simulink library "NFSModelsLibrary"  (R2020a)
settings: Solver=VariableStepAuto  StartTime=0.0  StopTime=10.0  RelTol=1e-3
undefined symbols (not defined in the file or in its folder): Earth, F, Light, MIL, Newton, nfs, Raphson, sigbuilder_block, WGS84
libraries: sharedutil x3, simulink x2, ModelsLibrary x2, $bdroot x2, aerolibwind2 x2, aerolibtransform2 x1
(part 1 of 3)
settings Model: Creator=AHKh  LastModifiedBy=AHKh
settings DataIOCC: ReturnWorkspaceOutputs=off
settings DebuggingCC: ArithmeticOperatorsInVariantConditions=warning
settings SFSimCC: SimUseLocalCustomCode=off  CustomCodeUndefinedFunction=UseInterfaceOnly
settings RTWCC: RTWUseLocalCustomCode=off
settings CodeAppCC: StateflowObjectComments=on

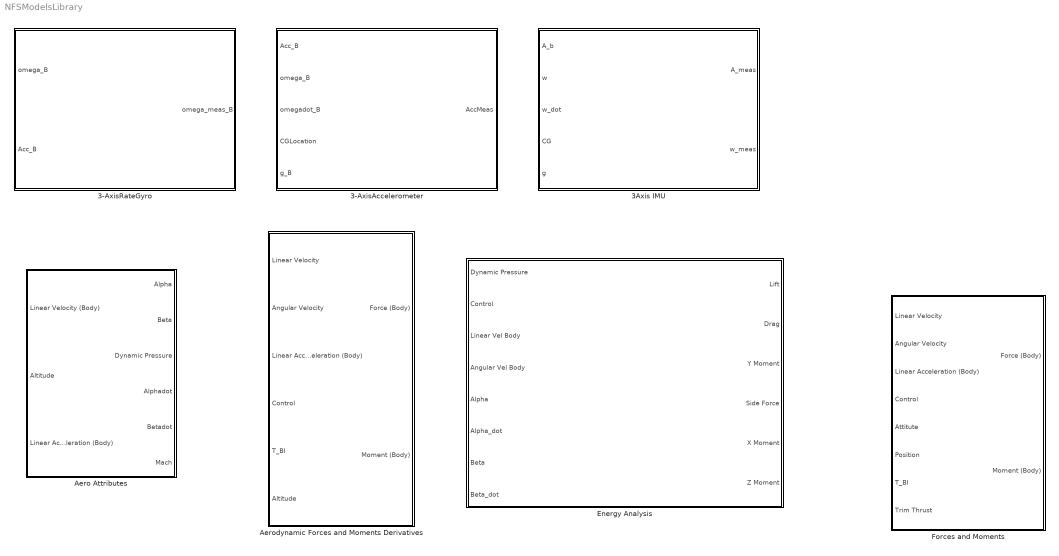
== system NFSModelsLibrary ==
  3-AxisAccelerometer : Subsystem  mask{units=Metric (MKS), SensorLoc=[0; 0; 0], gtype=off, dtype_a=on, w_a=190, z_a=0.707, SFCC=eye(3), SensorBias=[0; 0; 0], Ts=0.001, AccNoiseCheck=on, NoiseSeeds=[23093; 23094; 23095], NoisePower=[0.001; 0.001; 0.001], satUpper=[inf; inf; inf], satLower=[-inf; -inf; -inf]}
      mask prompts: units "Unit"; SensorLoc "Accelerometer Location"; gtype "Subtracting Gravity"; dtype_a "Considering 2nd-Order Dynamics"; w_a "Natural Frequency (rad/s)"; z_a "Damping Ratio"; SFCC "Scale Factor and Cross-Coupling"; SensorBias "Measurment Bias"; Ts "Update Rate (sec)"; AccNoiseCheck "Considering Noise"; NoiseSeeds "Noise Seeds"; NoisePower "Noise Power"; satUpper "Output Upper Limits"; satLower "Output Lower Limits"
      mask TypeOptions units: Metric (MKS)
      mask DialogControl DescGroupVar Prompt: Three-Axis Accelerometer
      mask DialogControl DescTextVar Prompt: Implements a three-axis accelerometer
      mask DialogControl Container4 Prompt: Main
      mask DialogControl units Tooltip: Metric System of Units
      mask DialogControl Container5 Prompt: Noise Characteristics
      mask Display:
      | port_label('input',1,'[Acc]^{B}_B (m/s^2)','texmode','on');
      | port_label('input',2,'[\omega]^B_B (rad/s)','texmode','on');
      | port_label('input',3,'[d\omega/dt]^B_B (rad/s^2)','texmode','on');
      | port_label('input',4,'[CG]^B_B (m)','texmode','on');
      | port_label('input',5,'[g]^B_B (m/s^2)','texmode','on');
      | port_label('output',1,'[Acc_{meas}]^{B}_B (m/s^2)','texmode','on');
  3-AxisRateGyro : Subsystem  mask(Three-Axis Rate Gyroscope){dtype_g=on, w_g=190, z_g=0.707, SFCC=eye(3), SensorBias=[0; 0; 0], gSensitivity=[0; 0; 0], Ts=0.001, GyroNoiseCheck=on, NoiseSeeds=[23093; 23094; 23095], NoisePower=[0.0001; 0.0001; 0.0001], satUpper=[inf; inf; inf], satLower=[-inf; -inf; -inf]}
      mask prompts: dtype_g "Considering 2nd-Order Dynamics"; w_g "Natural Frequency (rad/s)"; z_g "Damping Ratio"; SFCC "Scale Factors and Cross-Coupling"; SensorBias "Measurment Bias"; gSensitivity "G-Sensitive Bias"; Ts "Update Rate (sec)"; GyroNoiseCheck "Considering Noise"; NoiseSeeds "Noise Seeds"; NoisePower "Noise Power"; satUpper "Output Upper Bound"; satLower "Output Lower Bound"
      mask DialogControl DescGroupVar Prompt: Three-Axis Gyroscope
      mask DialogControl DescTextVar Prompt: Implements a three-axis gyroscope.
      mask DialogControl Container4 Prompt: Main
      mask DialogControl Container5 Prompt: Noise Characteristics
      mask Display:
      | port_label('input',1,'[\omega]^B_B (rad/s)','texmode','on');
      | port_label('input',2,'[Acc]^{B}_B (m/s^2)','texmode','on');
      | port_label('output',1,'[\omega_{meas}]^{B}_B (rad/s)','texmode','on');
  3Axis IMU : Subsystem  mask{units=Metric (MKS), IMULocation=[0; 0; 0], Ts=0.001, AccSubtractGravity=off, dtype_a=on, AccNaturalFrequency=190, AccDampingRatio=0.707, AccSFCC=eye(3), AccMeasurmentBias=[0; 0; 0], AccMeasUpperLimit=[inf; inf; inf], AccMeasLowerLimit=[-inf; -inf; -inf], AccNoiseCheck=on, AccNoiseSeeds=[23093; 23094; 23095], AccNoisePower=[0.0001; 0.0001; 0.0001], dtype_g=on, GyroNaturalFrequency=190, GyroDampingRatio=0.707, GyroSFCC=eye(3), GyroMeasurmentBias=[0; 0; 0], GyroGSensitiveBias=[0; 0; 0], GyroMeasUpperLimit=[inf; inf; inf], GyroMeasLowerLimit=[-inf; -inf; -inf], GyroNoiseCheck=on, GyroNoiseSeeds=[23093; 23094; 23095], GyroNoisePower=[0.0001; 0.0001; 0.0001]}
      mask prompts: IMULocation "IMU Location (m)"; Ts "Update Rate (sec)"; AccSubtractGravity "Subtracting Gravity"; dtype_a "Considering 2nd-Order Dynamics"; AccNaturalFrequency "Natural Frequency (rad/s)"; AccDampingRatio "Damping Ratio"; AccSFCC "Scale Factor and Cross Coupling"; AccMeasurmentBias "Measurment Bias"; AccMeasUpperLimit "Measurment Upper Limit"; AccMeasLowerLimit "Measurment Lower Limit"; AccNoiseCheck "Considering Noise"; AccNoiseSeeds "Noise Seeds"; AccNoisePower "Noise Power"; dtype_g "Considering 2nd-Order Dynamics"; GyroNaturalFrequency "Natural Frequency (rad/s)"; GyroDampingRatio "Damping Ratio"; GyroSFCC "Scale Factor and Cross Coupling"; GyroMeasurmentBias "Measurment Bias"; GyroGSensitiveBias "G-Sensitive Bias"; GyroMeasUpperLimit "Measurment Upper Limit"; GyroMeasLowerLimit "Measurment Lower Limit"; GyroNoiseCheck "Considering Noise"; GyroNoiseSeeds "Noise Seeds"; GyroNoisePower "Noise Power"
      mask init:
      | a1 = get(gcbh,'AccSubtractGravity');
      | a2 = get(gcbh,'dtype_a');
      | a3 = get(gcbh,'AccNoiseCheck');
      | a4 = get(gcbh,'dtype_g');
      | a5 = get(gcbh,'GyroNoiseCheck');
      | Acc = getSimulinkBlockHandle([gcb '/3-AxisAccelerometer']);
      | Gyro = getSimulinkBlockHandle([gcb '/3-AxisRateGyro']);
      | set(Acc,'gtype',a1);
      | set(Acc,'dtype_a',a2);
      | set(Acc,'AccNoiseCheck',a3);
      | set(Gyro,'dtype_g',a4);
      | set(Gyro,'GyroNoiseCheck',a5);
      mask TypeOptions units: Metric (MKS)
      mask DialogControl DescGroupVar Prompt: 3-Axis IMU
      mask DialogControl DescTextVar Prompt: Implements 3-axis Inertial Measurment Unit (IMU)
      mask DialogControl Container4 Prompt: Main
      mask DialogControl Container9 Prompt: Accelerometer
      mask DialogControl Container11 Prompt: Accelerometer General
      mask DialogControl Container14 Prompt: Accelerometer Noise
      mask DialogControl Container5 Prompt: Gyroscope
      mask DialogControl Container7 Prompt: Gyroscope General
      mask DialogControl Container8 Prompt: Gyroscope Noise
      mask Display:
      | port_label('input',1,'[Acc]^{B}_B (m/s^2)','texmode','on');
      | port_label('input',2,'[\omega]^B_B (rad/s)','texmode','on');
      | port_label('input',3,'[d\omega/dt]^B_B (rad/s^2)','texmode','on');
      | port_label('input',4,'[CG]^B_B (m)','texmode','on');
      | port_label('input',5,'[g]^B_B (m/s^2)','texmode','on');
      | port_label('output',1,'[Acc_{meas}]^{B}_B (m/s^2)','texmode','on');
      | port_label('output',2,'[\omega_{meas}]^{B}_B (rad/s)','texmode','on');
  Aero Attributes : Subsystem
  Aerodynamic Forces and Moments Derivatives : Subsystem
  Energy Analysis : Subsystem  mask{ae=nfs}
      mask prompts: ae "Aero Coefficients"
  Forces and Moments : Subsystem

== system NFSModelsLibrary/3-AxisAccelerometer ==
  Acc_B : Inport  Unit=m/s^2  PortDimensions=[3,1]
  omega_B : Inport  Port=2  Unit=rad/s  PortDimensions=[3,1]
  omegadot_B : Inport  Port=3  Unit=rad/s^2  PortDimensions=[3,1]
  CGLocation : Inport  Port=4  Unit=m  PortDimensions=[3,1]
  g_B : Inport  Port=5  Unit=m/s^2  PortDimensions=[3,1]
  Accelerometer Dynamic : Subsystem
  Gain : Gain  Gain=[1 -1 1]'  SaturateOnIntegerOverflow=on  OutDataTypeStr=Inherit: Same as input  ParamDataTypeStr=Inherit: Same as input
  Measurement bias : Constant  Value=SensorBias
  Noise Check : Subsystem
  Product : Product  Multiplication=Matrix(*)  SaturateOnIntegerOverflow=on  OutDataTypeStr=Inherit: Same as first input
  Random bias : simulink/Sources/Band-Limited White Noise  Cov=NoisePower  Ts=Ts  seed=NoiseSeeds
  Reshape : Reshape  OutputDimensionality=Column vector (2-D)
  Reshape1 : Reshape
  Saturation : Saturate  UpperLimit=satUpper  LowerLimit=satLower
  Scale factors & Cross-coupling errors : Constant  Value=SFCC
  Sum1 : Sum  Inputs=|++  SaturateOnIntegerOverflow=on
  Sum2 : Sum  Inputs=|+-
  Sum3 : Sum  Inputs=|++
  Sum4 : Sum  Inputs=++|  SaturateOnIntegerOverflow=on
  Sum5 : Sum  Inputs=|++
  Sum7 : Sum  Inputs=|+-  SaturateOnIntegerOverflow=on
  w x (w x d) : Subsystem
  wdot x d : sharedutil/3x3 Cross Product
      settings: SourceProductBaseCode=AE,PW,MT,VE,VP
  wl_ins : Constant  Value=SensorLoc
  AccMeas : Outport  Unit=m/s^2  PortDimensions=[3,1]  VectorParamsAs1DForOutWhenUnconnected=off
  wires:
  Gain/1 -> w x (w x d)/2(CGAccdistance), wdot x d/2
  Sum4/1 -> Accelerometer Dynamic/1(AccIn)
  omegadot_B/1 -> wdot x d/1
  omega_B/1 -> w x (w x d)/1(omega_B)
  Scale factors & Cross-coupling errors/1 -> Product/1
  Measurement bias/1 -> Sum4/2
  Sum7/1 -> Gain/1
  wdot x d/1 -> Sum5/2
  CGLocation/1 -> Sum7/1
  Accelerometer Dynamic/1("AccOut ") -> Sum1/1
  Saturation/1 -> AccMeas/1
  Product/1 -> Reshape1/1
  Sum1/1 -> Saturation/1
  Random bias/1 -> Noise Check/1(NoiseIn)
  Reshape1/1 -> Sum4/1
  Sum5/1 -> Product/2
  Acc_B/1 -> Sum2/1
  g_B/1 -> Sum2/2
  Sum2/1 -> Sum3/1
  w x (w x d)/1(w x ( w x d)) -> Sum3/2
  Sum3/1 -> Sum5/1
  wl_ins/1 -> Reshape/1
  Reshape/1 -> Sum7/2
  Noise Check/1("NoiseOut ") -> Sum1/2

== system NFSModelsLibrary/3-AxisRateGyro ==
  omega_B : Inport  Unit=rad/s  PortDimensions=3
  Acc_B : Inport  Port=2  Unit=m/s^2  PortDimensions=3
  Gravity : Constant  Value=9.806
  Gyroscope Dynamic : Subsystem
  Measurement bias : Constant  Value=SensorBias
  Noise Check : Subsystem
  Product : Product  Multiplication=Matrix(*)  SaturateOnIntegerOverflow=on  OutDataTypeStr=Inherit: Same as first input
  Product1 : Product  SaturateOnIntegerOverflow=on  OutDataTypeStr=Inherit: Same as first input
  Product2 : Product  Inputs=*/  SaturateOnIntegerOverflow=on  OutDataTypeStr=Inherit: Same as first input
  Random bias : simulink/Sources/Band-Limited White Noise  Cov=NoisePower  Ts=Ts  seed=NoiseSeeds
  Saturation : Saturate  UpperLimit=satUpper  LowerLimit=satLower
  "Scale factors & Cross-coupling errors " : Constant  Value=SFCC
  Sum1 : Sum  Inputs=|++  SaturateOnIntegerOverflow=on
  Sum4 : Sum  Inputs=+++  SaturateOnIntegerOverflow=on
  g-sensitive bias : Constant  Value=gSensitivity
  omega_meas_B : Outport  Unit=rad/s  VectorParamsAs1DForOutWhenUnconnected=off
  wires:
  Product/1 -> Sum4/1
  Gyroscope Dynamic/1(pqr Out) -> Sum1/1
  Acc_B/1 -> Product2/1
  Product2/1 -> Product1/1
  Sum1/1 -> Saturation/1
  omega_B/1 -> Product/2
  Random bias/1 -> Noise Check/1(NoiseIn)
  Saturation/1 -> omega_meas_B/1
  Measurement bias/1 -> Sum4/2
  "Scale factors & Cross-coupling errors "/1 -> Product/1
  Sum4/1 -> Gyroscope Dynamic/1(pqr In)
  g-sensitive bias/1 -> Product1/2
  Product1/1 -> Sum4/3
  Gravity/1 -> Product2/2
  Noise Check/1("NoiseOut ") -> Sum1/2

== system NFSModelsLibrary/3Axis IMU ==
  A_b : Inport  Unit=m/s^2  PortDimensions=[3,1]
  w : Inport  Port=2  Unit=rad/s  PortDimensions=[3,1]
  w_dot : Inport  Port=3  Unit=rad/s^2  PortDimensions=[3,1]
  CG : Inport  Port=4  Unit=m  PortDimensions=[3,1]
  g : Inport  Port=5  Unit=m/s^2  PortDimensions=[3,1]
  3-AxisAccelerometer : ModelsLibrary/3-AxisAccelerometer  units=Metric (MKS)  SensorLoc=IMULocation  gtype=off  dtype_a=on  w_a=AccNaturalFrequency  z_a=AccDampingRatio  SFCC=AccSFCC  SensorBias=AccMeasurmentBias  Ts=Ts  AccNoiseCheck=on  NoiseSeeds=AccNoiseSeeds  NoisePower=AccNoisePower  satUpper=AccMeasUpperLimit  satLower=AccMeasLowerLimit
  3-AxisRateGyro : ModelsLibrary/3-AxisRateGyro  dtype_g=on  w_g=GyroNaturalFrequency  z_g=GyroDampingRatio  SFCC=GyroSFCC  SensorBias=GyroMeasurmentBias  gSensitivity=GyroGSensitiveBias  Ts=Ts  GyroNoiseCheck=on  NoiseSeeds=GyroNoiseSeeds  NoisePower=GyroNoisePower  satUpper=GyroMeasUpperLimit  satLower=GyroMeasLowerLimit
  A_meas : Outport  Unit=m/s^2  PortDimensions=[3,1]  VectorParamsAs1DForOutWhenUnconnected=off
  w_meas : Outport  Port=2  Unit=rad/s  PortDimensions=[3,1]  VectorParamsAs1DForOutWhenUnconnected=off
  wires:
  3-AxisRateGyro/1 -> w_meas/1
  w/1 -> 3-AxisRateGyro/1, 3-AxisAccelerometer/2
  A_b/1 -> 3-AxisRateGyro/2, 3-AxisAccelerometer/1
  3-AxisAccelerometer/1 -> A_meas/1
  w_dot/1 -> 3-AxisAccelerometer/3
  CG/1 -> 3-AxisAccelerometer/4
  g/1 -> 3-AxisAccelerometer/5

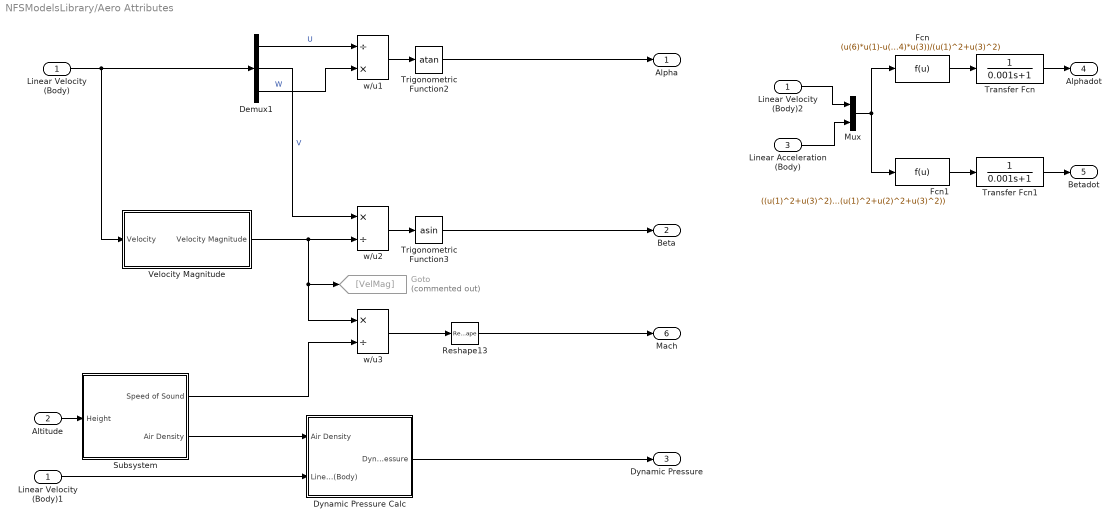
== system NFSModelsLibrary/Aero Attributes ==
  Linear Velocity (Body) : Inport  PortDimensions=[3,1]
  Altitude : Inport  Port=2
  Linear Acceleration (Body) : Inport  Port=3  PortDimensions=[3,1]
  Demux1 : Demux  Outputs=3
      settings: DisplayOption=none
  Dynamic Pressure Calc : Subsystem
  Fcn : Fcn  Expr=(u(6)*u(1)-u(4)*u(3))/(u(1)^2+u(3)^2)
  Fcn1 : Fcn  Expr=((u(1)^2+u(3)^2)*u(5)-u(2)*(u(1)*u(4)+u(3)*u(6)))/(sqrt(u(1)^2+u(3)^2)*(u(1)^2+u(2)^2+u(3)^2))
  Goto : Goto  Commented=on  GotoTag=VelMag
  Linear Velocity (Body)1 : InportShadow  PortDimensions=[3,1]
  Linear Velocity (Body)2 : InportShadow  PortDimensions=[3,1]
  Mux : Mux  Inputs=2
  Reshape13 : Reshape
  Subsystem : Subsystem
  Transfer Fcn : TransferFcn  Denominator=[0.001 1]
  Transfer Fcn1 : TransferFcn  Denominator=[0.001 1]
  Trigonometric Function2 : Trigonometry  Operator=atan
  Trigonometric Function3 : Trigonometry  Operator=asin
  Velocity Magnitude : Subsystem
  w/u1 : Product  Inputs=/*  InputSameDT=on  SaturateOnIntegerOverflow=on  OutDataTypeStr=Inherit: Same as first input
  w/u2 : Product  Inputs=*/  InputSameDT=on  SaturateOnIntegerOverflow=on  OutDataTypeStr=Inherit: Same as first input
  w/u3 : Product  Inputs=*/  InputSameDT=on  SaturateOnIntegerOverflow=on  OutDataTypeStr=Inherit: Same as first input
  Alpha : Outport  VectorParamsAs1DForOutWhenUnconnected=off
  Beta : Outport  Port=2  VectorParamsAs1DForOutWhenUnconnected=off
  Dynamic Pressure : Outport  Port=3  VectorParamsAs1DForOutWhenUnconnected=off
  Alphadot : Outport  Port=4  VectorParamsAs1DForOutWhenUnconnected=off
  Betadot : Outport  Port=5  VectorParamsAs1DForOutWhenUnconnected=off
  Mach : Outport  Port=6  VectorParamsAs1DForOutWhenUnconnected=off
  wires:
  Fcn1/1 -> Transfer Fcn1/1
  Fcn/1 -> Transfer Fcn/1
  Mux/1 -> Fcn/1, Fcn1/1
  Linear Acceleration (Body)/1 -> Mux/2
  Linear Velocity (Body)2/1 -> Mux/1
  Linear Velocity (Body)/1 -> Demux1/1, Velocity Magnitude/1(Velocity)
  Demux1/1 -> w/u1/1  "U"
  Demux1/2 -> w/u2/1  "V"
  Demux1/3 -> w/u1/2  "W"
  w/u1/1 -> Trigonometric Function2/1
  w/u2/1 -> Trigonometric Function3/1
  Trigonometric Function2/1 -> Alpha/1
  w/u3/1 -> Reshape13/1
  Altitude/1 -> Subsystem/1(Height)
  Linear Velocity (Body)1/1 -> Dynamic Pressure Calc/2(Linear Velocity (Body))
  Dynamic Pressure Calc/1(Dynamic Pressure) -> Dynamic Pressure/1
  Trigonometric Function3/1 -> Beta/1
  Reshape13/1 -> Mach/1
  Velocity Magnitude/1(Velocity Magnitude) -> w/u2/2, w/u3/1, Goto/1
  Subsystem/1(Speed of Sound) -> w/u3/2
  Subsystem/2(Air Density) -> Dynamic Pressure Calc/1(Air Density)
  Transfer Fcn/1 -> Alphadot/1
  Transfer Fcn1/1 -> Betadot/1

== system NFSModelsLibrary/Aerodynamic Forces and Moments Derivatives ==
  Linear Velocity : Inport
  Angular Velocity : Inport  Port=2
  Linear Acceleration (Body) : Inport  Port=3
  Control : Inport  Port=4
  T_BI : Inport  Port=5
  Altitude : Inport  Port=6
  Aero Attributes : $bdroot/Aero Attributes  SystemSampleTime=-1  Latency=0  AutoFrameSizeCalculation=off
  Bus Selector : BusSelector  OutputSignals=Linear Velocity,Angular Velocity
  Forces : Subsystem
  Moments : Subsystem
  Terminator : Terminator
  Turbulence : Subsystem
  Force (Body) : Outport  VectorParamsAs1DForOutWhenUnconnected=off
  Moment (Body) : Outport  Port=2  VectorParamsAs1DForOutWhenUnconnected=off
  wires:
  Linear Acceleration (Body)/1 -> Aero Attributes/3
  Turbulence/1(Turbulent Velocity) -> Bus Selector/1
  Angular Velocity/1 -> Turbulence/2(Angular Velocity)
  Bus Selector/2 -> Moments/4(Angular Velocity), Forces/4(Angular Velocity)  "<Angular Velocity>"
  Aero Attributes/3 -> Moments/6(Dynamic Pressure), Forces/6(Dynamic Pressure)
  Aero Attributes/1 -> Moments/2(Alpha), Forces/2(Alpha)
  Aero Attributes/4 -> Moments/7(Alphadot), Forces/7(Alphadot)
  Aero Attributes/2 -> Moments/3(Beta), Forces/3(Beta)
  Control/1 -> Moments/5(Control), Forces/5(Control)
  Aero Attributes/6 -> Forces/8(Mach), Moments/8(Mach)
  Linear Velocity/1 -> Turbulence/1(Linear Velocity)
  Aero Attributes/5 -> Terminator/1
  Forces/1(Aerodynamic Forces (Body)) -> Force (Body)/1
  Moments/1(Aerodynamic Moments (Body)) -> Moment (Body)/1
  Altitude/1 -> Aero Attributes/2, Turbulence/3(Altitude)
  T_BI/1 -> Turbulence/4(DCM)
  Bus Selector/1 -> Aero Attributes/1, Moments/1(Linear Velocity), Forces/1(Linear Velocity)  "<Linear Velocity>"

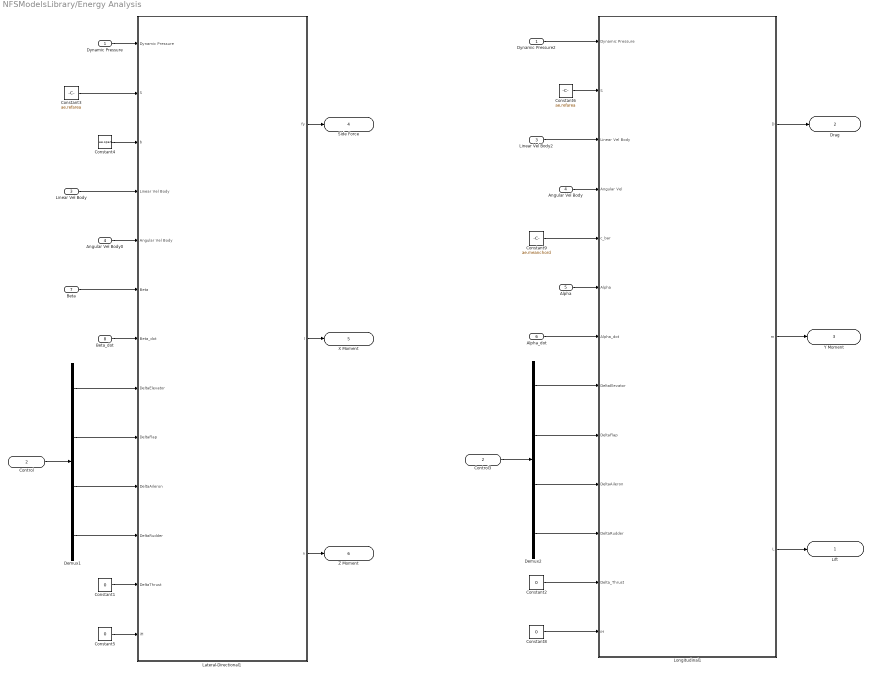
== system NFSModelsLibrary/Energy Analysis ==
  Dynamic Pressure : Inport
  Control : Inport  Port=2
  Linear Vel Body : Inport  Port=3
  Angular Vel Body : Inport  Port=4
  Alpha : Inport  Port=5
  Alpha_dot : Inport  Port=6
  Beta : Inport  Port=7
  Beta_dot : Inport  Port=8
  Angular Vel Body0 : InportShadow  Port=4
  Constant{1..2,5,8} (4 alike) : Constant  Value=0
  Constant3 : Constant  Value=ae.refarea
  Constant4 : Constant  Value=ae.span
  Constant6 : Constant  Value=ae.refarea
  Constant9 : Constant  Value=ae.meanchord
  Control3 : InportShadow  Port=2
  Demux1 : Demux
  Demux2 : Demux
  Dynamic Pressure2 : InportShadow
  Lateral-Directional1 : Subsystem
  Linear Vel Body2 : InportShadow  Port=3
  Longitudinal1 : Subsystem
  Lift : Outport  VectorParamsAs1DForOutWhenUnconnected=off
  Drag : Outport  Port=2  VectorParamsAs1DForOutWhenUnconnected=off
  Y Moment : Outport  Port=3  VectorParamsAs1DForOutWhenUnconnected=off
  Side Force : Outport  Port=4  VectorParamsAs1DForOutWhenUnconnected=off
  X Moment : Outport  Port=5  VectorParamsAs1DForOutWhenUnconnected=off
  Z Moment : Outport  Port=6  VectorParamsAs1DForOutWhenUnconnected=off
  wires:
  Lateral-Directional1/1(fy) -> Side Force/1
  Lateral-Directional1/2(l) -> X Moment/1
  Lateral-Directional1/3(n) -> Z Moment/1
  Longitudinal1/2(m) -> Y Moment/1
  Longitudinal1/1(D) -> Drag/1
  Longitudinal1/3(L) -> Lift/1
  Dynamic Pressure/1 -> Lateral-Directional1/1(Dynamic Pressure)
  Constant3/1 -> Lateral-Directional1/2(S)
  Linear Vel Body/1 -> Lateral-Directional1/4(Linear Vel Body)
  Angular Vel Body0/1 -> Lateral-Directional1/5(Angular Vel Body)
  Constant5/1 -> Lateral-Directional1/13(iH)
  Constant4/1 -> Lateral-Directional1/3(b)
  Beta/1 -> Lateral-Directional1/6(Beta)
  Beta_dot/1 -> Lateral-Directional1/7(Beta_dot)
  Demux1/1 -> Lateral-Directional1/8(DeltaElevator)
  Demux1/2 -> Lateral-Directional1/9(DeltaFlap)
  Demux1/4 -> Lateral-Directional1/11(DeltaRudder)
  Demux1/3 -> Lateral-Directional1/10(DeltaAileron)
  Constant1/1 -> Lateral-Directional1/12(DeltaThrust)
  Control/1 -> Demux1/1
  Constant6/1 -> Longitudinal1/2(S)
  Alpha/1 -> Longitudinal1/6(Alpha)
  Angular Vel Body/1 -> Longitudinal1/4(Angular Vel)
  Dynamic Pressure2/1 -> Longitudinal1/1(Dynamic Pressure)
  Linear Vel Body2/1 -> Longitudinal1/3(Linear Vel Body)
  Constant9/1 -> Longitudinal1/5(c_bar)
  Alpha_dot/1 -> Longitudinal1/7(Alpha_dot)
  Constant8/1 -> Longitudinal1/13(iH)
  Constant2/1 -> Longitudinal1/12(Delta_Thrust)
  Demux2/4 -> Longitudinal1/11(DeltaRudder)
  Demux2/2 -> Longitudinal1/9(DeltaFlap)
  Demux2/3 -> Longitudinal1/10(DeltaAileron)
  Demux2/1 -> Longitudinal1/8(DeltaElevator)
  Control3/1 -> Demux2/1

== system NFSModelsLibrary/Forces and Moments ==
  Linear Velocity : Inport
  Angular Velocity : Inport  Port=2
  Linear Acceleration (Body) : Inport  Port=3
  Control : Inport  Port=4
  Attitute : Inport  Port=5  PortDimensions=[3,1]
  Position : Inport  Port=6
  T_BI : Inport  Port=7
  Trim Thrust : Inport  Port=8
  Aerodynamic Forces and Moments Derivatives : $bdroot/Aerodynamic Forces and Moments Derivatives  SystemSampleTime=-1  Latency=0  AutoFrameSizeCalculation=off
  Gravity Calculator : Subsystem
  Sum{,1..3} (4 alike) : Sum  Inputs=|++
  Thrust : Subsystem
  Weight : Subsystem
  Force (Body) : Outport  VectorParamsAs1DForOutWhenUnconnected=off
  Moment (Body) : Outport  Port=2  VectorParamsAs1DForOutWhenUnconnected=off
  wires:
  [Altitude] -> Aerodynamic Forces and Moments Derivatives/6
  Attitute/1 -> Weight/1(Attitute)
  Position/1 -> Gravity Calculator/1(Position (NED))
  Gravity Calculator/2(Altitud) -> [Altitude]
  Sum2/1 -> Force (Body)/1
  Linear Velocity/1 -> Aerodynamic Forces and Moments Derivatives/1
  T_BI/1 -> Aerodynamic Forces and Moments Derivatives/5
  Weight/1(Weight Force) -> Sum2/2
  Aerodynamic Forces and Moments Derivatives/2 -> Sum1/1
  Sum1/1 -> Sum3/1
  Gravity Calculator/1(Gravity (NED)) -> [Gravity]
  Thrust/2(Thrust Moment) -> Sum1/2
  Aerodynamic Forces and Moments Derivatives/1 -> Sum/1
  Sum/1 -> Sum2/1
  Control/1 -> Aerodynamic Forces and Moments Derivatives/4
  Weight/2(Weight Moment) -> Sum3/2
  Sum3/1 -> Moment (Body)/1
  Angular Velocity/1 -> Aerodynamic Forces and Moments Derivatives/2
  Thrust/1(Thrust Force) -> Sum/2
  Linear Acceleration (Body)/1 -> Aerodynamic Forces and Moments Derivatives/3
  [Gravity] -> Weight/2(Gravity)
  Trim Thrust/1 -> Thrust/1(Trim Thrust)

== system NFSModelsLibrary/3-AxisAccelerometer/Accelerometer Dynamic ==
  AccIn : Inport
  Constant : Constant  Value=dtype_a
  No Dynamics : Subsystem
  Second-order Dynamics : Subsystem
  Switch : Switch  Threshold=0.5
  "AccOut " : Outport  VectorParamsAs1DForOutWhenUnconnected=off
  wires:
  Constant/1 -> Switch/2
  Switch/1 -> "AccOut "/1
  Second-order Dynamics/1("Out ") -> Switch/1
  AccIn/1 -> No Dynamics/1(In), Second-order Dynamics/1(In)
  No Dynamics/1("Out ") -> Switch/3

== system NFSModelsLibrary/3-AxisAccelerometer/Noise Check ==
  NoiseIn : Inport
  Constant : Constant  Value=AccNoiseCheck
  No Noise : Subsystem
  Noisy Signal : Subsystem
  Switch : Switch  Threshold=0.5
  "NoiseOut " : Outport  VectorParamsAs1DForOutWhenUnconnected=off
  wires:
  NoiseIn/1 -> No Noise/1(In), Noisy Signal/1(In)
  No Noise/1("Out ") -> Switch/3
  Noisy Signal/1("Out ") -> Switch/1
  Switch/1 -> "NoiseOut "/1
  Constant/1 -> Switch/2

== system NFSModelsLibrary/3-AxisAccelerometer/w x (w x d) ==
  omega_B : Inport  PortDimensions=[3,1]
  CGAccdistance : Inport  Port=2  PortDimensions=[3,1]
  w x (w x d) : sharedutil/3x3 Cross Product
      settings: SourceProductBaseCode=AE,PW,MT,VE,VP
  w x d : sharedutil/3x3 Cross Product
      settings: SourceProductBaseCode=AE,PW,MT,VE,VP
  w x ( w x d) : Outport  PortDimensions=[3,1]  VectorParamsAs1DForOutWhenUnconnected=off
  wires:
  w x d/1 -> w x (w x d)/2
  CGAccdistance/1 -> w x d/2
  omega_B/1 -> w x (w x d)/1, w x d/1
  w x (w x d)/1 -> w x ( w x d)/1

== system NFSModelsLibrary/3-AxisRateGyro/Gyroscope Dynamic ==
  pqr In : Inport  PortDimensions=[3,1]
  2nd-Order Dynamics : Subsystem
  Constant : Constant  Value=dtype_g
  No Dynamics : Subsystem
  Switch : Switch  Threshold=0.5
  pqr Out : Outport  SampleTime=[3,1]  VectorParamsAs1DForOutWhenUnconnected=off
  wires:
  pqr In/1 -> No Dynamics/1(In), 2nd-Order Dynamics/1(In)
  Constant/1 -> Switch/2
  No Dynamics/1(Out) -> Switch/3
  2nd-Order Dynamics/1(Out) -> Switch/1
  Switch/1 -> pqr Out/1

== system NFSModelsLibrary/3-AxisRateGyro/Noise Check ==
  NoiseIn : Inport
  Constant : Constant  Value=GyroNoiseCheck
  No Noise : Subsystem
  Noisy Signal : Subsystem
  Switch : Switch  Threshold=0.5
  "NoiseOut " : Outport  VectorParamsAs1DForOutWhenUnconnected=off
  wires:
  Constant/1 -> Switch/2
  Switch/1 -> "NoiseOut "/1
  Noisy Signal/1("Out ") -> Switch/1
  No Noise/1("Out ") -> Switch/3
  NoiseIn/1 -> Noisy Signal/1(In), No Noise/1(In)

== system NFSModelsLibrary/Aero Attributes/Dynamic Pressure Calc ==
  Air Density : Inport  PortDimensions=1
  Linear Velocity (Body) : Inport  Port=2  PortDimensions=[3 1]
  0.5*rh : Product  InputSameDT=on  SaturateOnIntegerOverflow=on  OutDataTypeStr=Inherit: Same as first input
  Dot Product : DotProduct  InputSameDT=on  OutDataTypeStr=Inherit: Inherit via internal rule
  Gain : Gain  Gain=0.5  SaturateOnIntegerOverflow=on  OutDataTypeStr=Inherit: Same as input  ParamDataTypeStr=Inherit: Same as input
  V^2 : Abs
  Dynamic Pressure : Outport  VectorParamsAs1DForOutWhenUnconnected=off
  wires:
  0.5*rh/1 -> Dynamic Pressure/1
  Gain/1 -> 0.5*rh/2
  V^2/1 -> 0.5*rh/1
  Air Density/1 -> Gain/1
  Linear Velocity (Body)/1 -> Dot Product/1, Dot Product/2
  Dot Product/1 -> V^2/1

== system NFSModelsLibrary/Aero Attributes/Subsystem ==
  Height : Inport
  "(T/T0)^(g/LR) " : Math  Operator=pow  SignedPower=on  SaturateOnIntegerOverflow=on
  1/T0 : Gain  Gain=1/288.15  SaturateOnIntegerOverflow=on  OutDataTypeStr=Inherit: Same as input  ParamDataTypeStr=Inherit: Same as input
  Altitude of Troposphere : Constant  Value=11000  OutDataTypeStr=Inherit: Inherit via back propagation
  Lapse Rate : Gain  Gain=0.0065  SaturateOnIntegerOverflow=on  OutDataTypeStr=Inherit: Same as input  ParamDataTypeStr=Inherit: Same as input
  Limit altitude  to Stratosphere : Saturate  UpperLimit=0  LowerLimit=11000-20000
  Limit altitude  to troposhere : Saturate  UpperLimit=11000  LowerLimit=0
  Product : Product  Inputs=*/  InputSameDT=on  SaturateOnIntegerOverflow=on  OutDataTypeStr=Inherit: Same as first input
  Product1 : Product  Inputs=/*  InputSameDT=on  SaturateOnIntegerOverflow=on  OutDataTypeStr=Inherit: Same as first input
  Product3 : Product  InputSameDT=on  SaturateOnIntegerOverflow=on  OutDataTypeStr=Inherit: Same as first input
  Sea Level Temperature : Constant  Value=288.15  OutDataTypeStr=Inherit: Inherit via back propagation
  Stratosphere Model : Math  SignedPower=on  SaturateOnIntegerOverflow=on
  Sum : Sum  Inputs=+-  InputSameDT=on  SaturateOnIntegerOverflow=on  OutDataTypeStr=Inherit: Same as first input
  Sum1 : Sum  Inputs=+-  InputSameDT=on  SaturateOnIntegerOverflow=on  OutDataTypeStr=Inherit: Same as first input
  a : Sqrt  AlgorithmType=Newton-Raphson  SaturateOnIntegerOverflow=on
  g/(L*R) : Constant  Value=9.80665/(0.0065*287.0531)  OutDataTypeStr=Inherit: Inherit via back propagation
  g/R : Gain  Gain=9.80665/287.0531  SaturateOnIntegerOverflow=on  OutDataTypeStr=Inherit: Same as input  ParamDataTypeStr=Inherit: Same as input
  gamma*R : Gain  Gain=1.4*287.0531  SaturateOnIntegerOverflow=on  OutDataTypeStr=Inherit: Same as input  ParamDataTypeStr=Inherit: Same as input
  rho0 : Gain  Gain=1.225  SaturateOnIntegerOverflow=on  OutDataTypeStr=Inherit: Same as input  ParamDataTypeStr=Inherit: Same as input
  Speed of Sound : Outport  PortDimensions=1  VectorParamsAs1DForOutWhenUnconnected=off
  Air Density : Outport  Port=2  PortDimensions=1  VectorParamsAs1DForOutWhenUnconnected=off
  wires:
  Limit altitude  to Stratosphere/1 -> g/R/1
  Sum/1 -> Limit altitude  to Stratosphere/1
  Altitude of Troposphere/1 -> Sum/1
  Product1/1 -> Stratosphere Model/1
  g/R/1 -> Product1/2
  Stratosphere Model/1 -> Product3/2
  Product3/1 -> Air Density/1
  rho0/1 -> Product3/1
  Sea Level Temperature/1 -> Sum1/1
  Lapse Rate/1 -> Sum1/2
  Sum1/1 -> Product1/1, 1/T0/1, gamma*R/1
  a/1 -> Speed of Sound/1
  gamma*R/1 -> a/1
  1/T0/1 -> Product/2, "(T/T0)^(g/LR) "/1
  "(T/T0)^(g/LR) "/1 -> Product/1
  Product/1 -> rho0/1
  Limit altitude  to troposhere/1 -> Lapse Rate/1
  Height/1 -> Sum/2, Limit altitude  to troposhere/1
  g/(L*R)/1 -> "(T/T0)^(g/LR) "/2

== system NFSModelsLibrary/Aero Attributes/Velocity Magnitude ==
  Velocity : Inport
  Dot Product : DotProduct  InputSameDT=on  OutDataTypeStr=Inherit: Inherit via internal rule
  Sqrt : Sqrt  SaturateOnIntegerOverflow=on
  Velocity Magnitude : Outport  VectorParamsAs1DForOutWhenUnconnected=off
  wires:
  Dot Product/1 -> Sqrt/1
  Velocity/1 -> Dot Product/1, Dot Product/2
  Sqrt/1 -> Velocity Magnitude/1  "abs(V)"

== system NFSModelsLibrary/Aerodynamic Forces and Moments Derivatives/Forces ==
  Linear Velocity : Inport  PortDimensions=[3,1]
  Alpha : Inport  Port=2  PortDimensions=1
  Beta : Inport  Port=3
  Angular Velocity : Inport  Port=4  PortDimensions=[3,1]
  Control : Inport  Port=5  PortDimensions=[4,1]
  Dynamic Pressure : Inport  Port=6  PortDimensions=[1,1]
  Alphadot : Inport  Port=7  PortDimensions=1
  Mach : Inport  Port=8
  Aerodynamic Forces : Subsystem
  Alpha1 : InportShadow  Port=2  PortDimensions=1
  Beta1 : InportShadow  Port=3
  Force Coefficients Calculator : Subsystem
  Aerodynamic Forces (Body) : Outport  VectorParamsAs1DForOutWhenUnconnected=off
  wires:
  Beta1/1 -> Aerodynamic Forces/6(Beta)
  Dynamic Pressure/1 -> Aerodynamic Forces/4(Dynamic Pressure)
  Alpha1/1 -> Aerodynamic Forces/5(Alpha)
  Force Coefficients Calculator/3(CY) -> Aerodynamic Forces/3(CY)
  Force Coefficients Calculator/2(CD) -> Aerodynamic Forces/2(CD)
  Force Coefficients Calculator/1(CL) -> Aerodynamic Forces/1(CL)
  Beta/1 -> Force Coefficients Calculator/3(Beta)
  Alpha/1 -> Force Coefficients Calculator/2(Alpha)
  Linear Velocity/1 -> Force Coefficients Calculator/1(Linear Velocity)
  Mach/1 -> Force Coefficients Calculator/7(Mach)
  Alphadot/1 -> Force Coefficients Calculator/6(Alphadot)
  Angular Velocity/1 -> Force Coefficients Calculator/4(Angular Velocity)
  Control/1 -> Force Coefficients Calculator/5(Control)
  Aerodynamic Forces/1(Aerodynamic Forces) -> Aerodynamic Forces (Body)/1

== system NFSModelsLibrary/Aerodynamic Forces and Moments Derivatives/Moments ==
  Linear Velocity : Inport  PortDimensions=[3,1]
  Alpha : Inport  Port=2
  Beta : Inport  Port=3
  Angular Velocity : Inport  Port=4  PortDimensions=[3,1]
  Control : Inport  Port=5
  Dynamic Pressure : Inport  Port=6
  Alphadot : Inport  Port=7
  Mach : Inport  Port=8
  "Aerodynamic Moment " : Subsystem
  Alpha1 : InportShadow  Port=2
  Beta1 : InportShadow  Port=3
  Beta2 : InportShadow  Port=3
  Demux1 : Demux  Outputs=3
      settings: DisplayOption=none
  Demux2 : Demux
      settings: DisplayOption=none
  Linear Velocity1 : InportShadow  PortDimensions=[3,1]
  Linear Velocity2 : InportShadow  PortDimensions=[3,1]
  Pitch Moment Coefficient : Subsystem
  Roll Moment Coefficient : Subsystem
  Yaw Moment Coefficient : Subsystem
  Aerodynamic Moments (Body) : Outport  VectorParamsAs1DForOutWhenUnconnected=off
  wires:
  Beta2/1 -> "Aerodynamic Moment "/6(Beta)
  Alpha1/1 -> "Aerodynamic Moment "/5(Alpha)
  Roll Moment Coefficient/1(Cl) -> "Aerodynamic Moment "/1(Cl)
  Pitch Moment Coefficient/1(Cm) -> "Aerodynamic Moment "/2(Cm)
  Yaw Moment Coefficient/1(Cn) -> "Aerodynamic Moment "/3(Cn)
  "Aerodynamic Moment "/1(Aerodynamic Moments) -> Aerodynamic Moments (Body)/1
  Linear Velocity/1 -> Roll Moment Coefficient/1(Linear Velocity)
  Linear Velocity1/1 -> Pitch Moment Coefficient/1(Linear Velocity)
  Linear Velocity2/1 -> Yaw Moment Coefficient/1(Linear Velocity)
  Dynamic Pressure/1 -> "Aerodynamic Moment "/4(Dynamic Pressure)
  Alpha/1 -> Pitch Moment Coefficient/2(Alpha)
  Beta/1 -> Roll Moment Coefficient/2(Beta)
  Beta1/1 -> Yaw Moment Coefficient/2(beta)
  Angular Velocity/1 -> Demux1/1
  Demux1/1 -> Roll Moment Coefficient/3(P), Yaw Moment Coefficient/3(P)
  Demux1/3 -> Roll Moment Coefficient/4(R), Yaw Moment Coefficient/4(R)
  Demux1/2 -> Pitch Moment Coefficient/3(Q)
  Alphadot/1 -> Pitch Moment Coefficient/6(Alphadot)
  Mach/1 -> Pitch Moment Coefficient/7(Mach)
  Control/1 -> Demux2/1
  Demux2/3 -> Roll Moment Coefficient/5(DeltaAileron), Yaw Moment Coefficient/5(DeltaAileron)
  Demux2/4 -> Roll Moment Coefficient/6(DeltaRudder), Yaw Moment Coefficient/6(DeltaRudder)
  Demux2/1 -> Pitch Moment Coefficient/4(DeltaElevator)
  Demux2/2 -> Pitch Moment Coefficient/5(DeltaFlap)

== system NFSModelsLibrary/Aerodynamic Forces and Moments Derivatives/Turbulence ==
  Linear Velocity : Inport  PortDimensions=[3,1]
  Angular Velocity : Inport  Port=2  PortDimensions=[3,1]
  Altitude : Inport  Port=3  PortDimensions=1
  DCM : Inport  Port=4  PortDimensions=[3,3]
  Bus Creator : BusCreator  Inputs=4
  Turbulence Model : Subsystem  Variant=on
  Turbulent Velocity : Outport  VectorParamsAs1DForOutWhenUnconnected=off
  wires:
  Turbulence Model/1(Out) -> Turbulent Velocity/1
  Angular Velocity/1 -> Bus Creator/2  "Angular Velocity"
  Bus Creator/1 -> Turbulence Model/1(In)
  DCM/1 -> Bus Creator/4  "DCM"
  Altitude/1 -> Bus Creator/3  "Altitude"
  Linear Velocity/1 -> Bus Creator/1  "Linear Velocity"

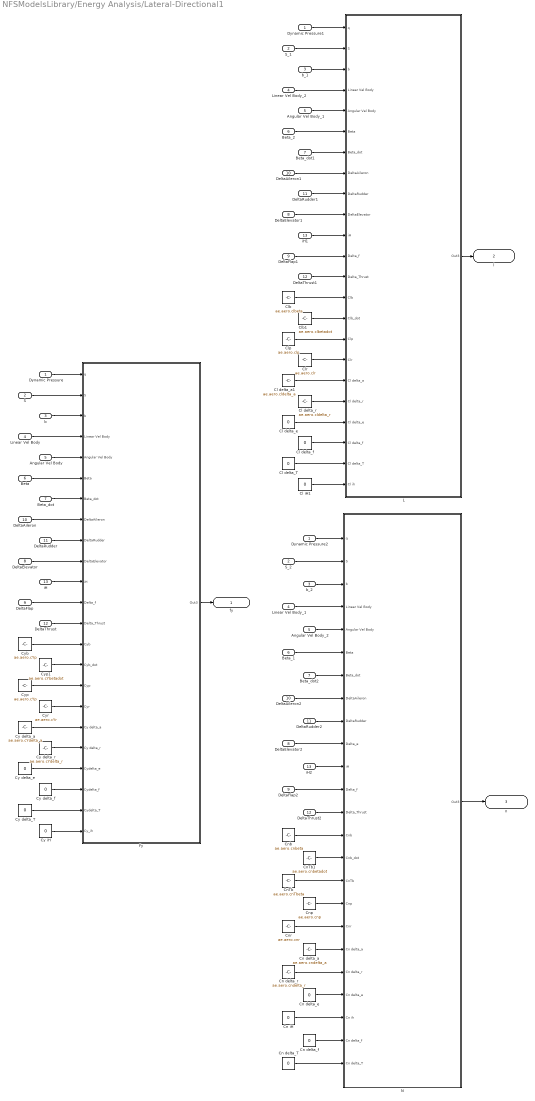
== system NFSModelsLibrary/Energy Analysis/Lateral-Directional1 ==
  Dynamic Pressure : Inport
  S : Inport  Port=2
  b : Inport  Port=3
  Linear Vel Body : Inport  Port=4
  Angular Vel Body : Inport  Port=5
  Beta : Inport  Port=6
  Beta_dot : Inport  Port=7
  DeltaElevator : Inport  Port=8
  DeltaFlap : Inport  Port=9
  DeltaAileron : Inport  Port=10
  DeltaRudder : Inport  Port=11
  DeltaThrust : Inport  Port=12
  iH : Inport  Port=13
  Angular Vel Body_1 : InportShadow  Port=5
  Angular Vel Body_2 : InportShadow  Port=5
  Beta_1 : InportShadow  Port=6
  Beta_2 : InportShadow  Port=6
  Beta_dot1 : InportShadow  Port=7
  Beta_dot2 : InportShadow  Port=7
  Cl delta_T : Constant  Value=0
  Cl delta_a1 : Constant  Value=ae.aero.cldelta_a
  Cl delta_e : Constant  Value=0
  Cl delta_f : Constant  Value=0
  Cl delta_r : Constant  Value=ae.aero.cldelta_r
  Cl iH1 : Constant  Value=0
  Clb : Constant  Value=ae.aero.clbeta
  Clb1 : Constant  Value=ae.aero.clbetadot
  Clp : Constant  Value=ae.aero.clp
  Clr : Constant  Value=ae.aero.clr
  Cn delta_T : Constant  Value=0
  Cn delta_a : Constant  Value=ae.aero.cndelta_a
  Cn delta_e : Constant  Value=0
  Cn delta_f : Constant  Value=0
  Cn delta_r : Constant  Value=ae.aero.cndelta_r
  Cn iH : Constant  Value=0
  CnTb : Constant  Value=ae.aero.cnTbeta
  CnTb1 : Constant  Value=ae.aero.cnbetadot
  Cnb : Constant  Value=ae.aero.cnbeta
  Cnp : Constant  Value=ae.aero.cnp
  Cnr : Constant  Value=ae.aero.cnr
  Cy delta_T : Constant  Value=0
  Cy delta_a : Constant  Value=ae.aero.cYdelta_a
  Cy delta_e : Constant  Value=0
  Cy delta_f : Constant  Value=0
  Cy delta_r : Constant  Value=ae.aero.cYdelta_r
  Cy iH : Constant  Value=0
  Cyb : Constant  Value=ae.aero.cYp
  Cyp : Constant  Value=ae.aero.cYp
  Cyp1 : Constant  Value=ae.aero.cYbetadot
  Cyr : Constant  Value=ae.aero.cYr
  DeltaAileron1 : InportShadow  Port=10
  DeltaAileron2 : InportShadow  Port=10
  DeltaElevator1 : InportShadow  Port=8
  DeltaElevator2 : InportShadow  Port=8
  DeltaFlap1 : InportShadow  Port=9
  DeltaFlap2 : InportShadow  Port=9
  DeltaRudder1 : InportShadow  Port=11
  DeltaRudder2 : InportShadow  Port=11
  DeltaThrust1 : InportShadow  Port=12
  DeltaThrust2 : InportShadow  Port=12
  Dynamic Pressure1 : InportShadow
  Dynamic Pressure2 : InportShadow
  Fy : Subsystem
  L : Subsystem
  Linear Vel Body_1 : InportShadow  Port=4
  Linear Vel Body_2 : InportShadow  Port=4
  N : Subsystem
  S_1 : InportShadow  Port=2
  S_2 : InportShadow  Port=2
  b_1 : InportShadow  Port=3
  b_2 : InportShadow  Port=3
  iH1 : InportShadow  Port=13
  iH2 : InportShadow  Port=13
  fy : Outport  VectorParamsAs1DForOutWhenUnconnected=off
  l : Outport  Port=2  VectorParamsAs1DForOutWhenUnconnected=off
  n : Outport  Port=3  VectorParamsAs1DForOutWhenUnconnected=off
  wires:
  L/1(Out3) -> l/1
  N/1(Out3) -> n/1
  Fy/1(Out3) -> fy/1
  Dynamic Pressure/1 -> Fy/1(q)
  S/1 -> Fy/2(S)
  b/1 -> Fy/3(b)
  Linear Vel Body/1 -> Fy/4(Linear Vel Body)
  Angular Vel Body/1 -> Fy/5(Angular Vel Body)
  Beta/1 -> Fy/6(Beta)
  Beta_dot/1 -> Fy/7(Beta_dot)
  DeltaAileron/1 -> Fy/8(DeltaAileron)
  DeltaRudder/1 -> Fy/9(DeltaRudder)
  iH/1 -> Fy/11(iH)
  DeltaElevator/1 -> Fy/10(DeltaElevator)
  DeltaFlap/1 -> Fy/12(Delta_f)
  DeltaThrust/1 -> Fy/13(Delta_Thrust)
  DeltaRudder2/1 -> N/9(DeltaRudder)
  DeltaAileron2/1 -> N/8(DeltaAileron)
  Dynamic Pressure2/1 -> N/1(q)
  DeltaThrust2/1 -> N/13(Delta_Thrust)
  b_2/1 -> N/3(b)
  Angular Vel Body_2/1 -> N/5(Angular Vel Body)
  Linear Vel Body_1/1 -> N/4(Linear Vel Body)
  iH2/1 -> N/11(iH)
  Beta_dot2/1 -> N/7(Beta_dot)
  S_2/1 -> N/2(S)
  DeltaElevator2/1 -> N/10(Delta_e)
  DeltaFlap2/1 -> N/12(Delta_f)
  Beta_1/1 -> N/6(Beta)
  Cyb/1 -> Fy/14(Cyb)
  Cyp/1 -> Fy/16(Cyp)
  Cyr/1 -> Fy/17(Cyr)
  Cy delta_a/1 -> Fy/18(Cy delta_a)
  Cy delta_r/1 -> Fy/19(Cy delta_r)
  Cy delta_e/1 -> Fy/20(Cydelta_e)
  Cy delta_f/1 -> Fy/21(Cydelta_f)
  Cy delta_T/1 -> Fy/22(Cydelta_T)
  Cy iH/1 -> Fy/23(Cy_ih)
  Cnb/1 -> N/14(Cnb)
  Cnp/1 -> N/17(Cnp)
  Cn delta_T/1 -> N/24(Cn delta_T)
  CnTb/1 -> N/16(CnTb)
  Cn delta_a/1 -> N/19(Cn delta_a)
  Cn delta_e/1 -> N/21(Cn delta_e)
  Cn delta_r/1 -> N/20(Cn delta_r)
  Cn iH/1 -> N/22(Cn ih)
  Cn delta_f/1 -> N/23(Cn delta_f)
  Cnr/1 -> N/18(Cnr)
  Clb/1 -> L/14(Clb)
  Clp/1 -> L/16(Clp)
  Cl delta_a1/1 -> L/18(Cl delta_a)
  b_1/1 -> L/3(b)
  Dynamic Pressure1/1 -> L/1(q)
  Angular Vel Body_1/1 -> L/5(Angular Vel Body)
  iH1/1 -> L/11(iH)
  DeltaRudder1/1 -> L/9(DeltaRudder)
  DeltaThrust1/1 -> L/13(Delta_Thrust)
  Beta_dot1/1 -> L/7(Beta_dot)
  Beta_2/1 -> L/6(Beta)
  DeltaAileron1/1 -> L/8(DeltaAileron)
  DeltaFlap1/1 -> L/12(Delta_f)
  DeltaElevator1/1 -> L/10(DeltaElevator)
  Linear Vel Body_2/1 -> L/4(Linear Vel Body)
  S_1/1 -> L/2(S)
  Clr/1 -> L/17(Clr)
  Cl delta_e/1 -> L/20(Cl delta_e)
  Cl delta_T/1 -> L/22(Cl delta_T)
  Cl delta_f/1 -> L/21(Cl delta_f)
  Cl delta_r/1 -> L/19(Cl delta_r)
  Cl iH1/1 -> L/23(Cl ih)
  Clb1/1 -> L/15(Clb_dot)
  CnTb1/1 -> N/15(Cnb_dot)
  Cyp1/1 -> Fy/15(Cyb_dot)

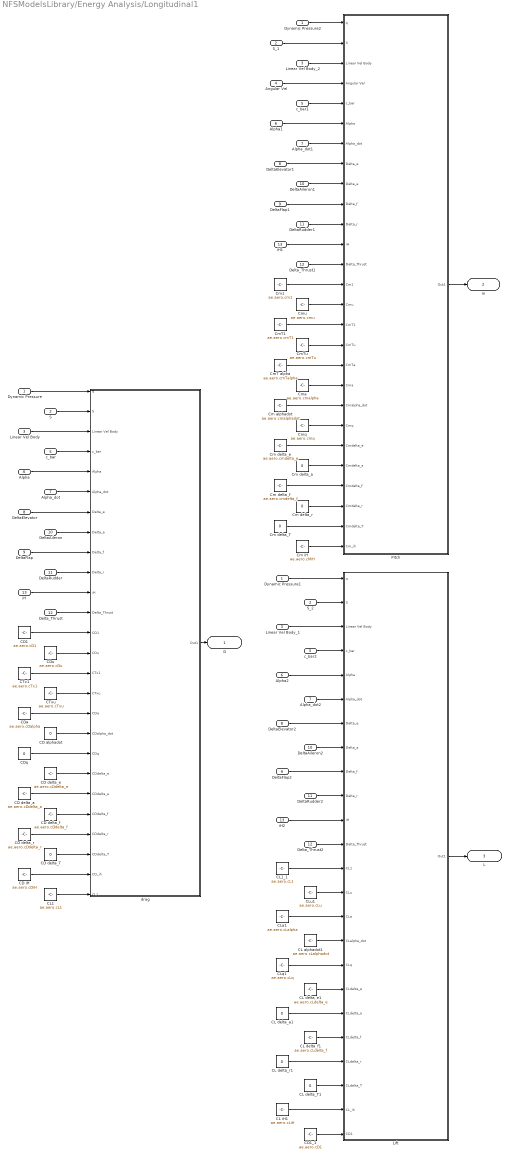
== system NFSModelsLibrary/Energy Analysis/Longitudinal1 ==
  Dynamic Pressure : Inport
  S : Inport  Port=2
  Linear Vel Body : Inport  Port=3
  Angular Vel : Inport  Port=4
  c_bar : Inport  Port=5
  Alpha : Inport  Port=6
  Alpha_dot : Inport  Port=7
  DeltaElevator : Inport  Port=8
  DeltaFlap : Inport  Port=9
  DeltaAileron : Inport  Port=10
  DeltaRudder : Inport  Port=11
  Delta_Thrust : Inport  Port=12
  iH : Inport  Port=13
  Alpha1 : InportShadow  Port=6
  Alpha2 : InportShadow  Port=6
  Alpha_dot1 : InportShadow  Port=7
  Alpha_dot2 : InportShadow  Port=7
  CD alphadot : Constant  Value=0
  CD delta_T : Constant  Value=0
  CD delta_a : Constant  Value=ae.aero.cDdelta_a
  CD delta_e : Constant  Value=ae.aero.cDdelta_e
  CD delta_f : Constant  Value=ae.aero.cDdelta_f
  CD delta_r : Constant  Value=ae.aero.cDdelta_r
  CD iH : Constant  Value=ae.aero.cDiH
  CD1 : Constant  Value=ae.aero.cD1
  CD1_1 : Constant  Value=ae.aero.cD1
  CDa : Constant  Value=ae.aero.cDalpha
  CDq : Constant  Value=0
  CDu : Constant  Value=ae.aero.cDu
  CL alphadot1 : Constant  Value=ae.aero.cLalphadot
  CL delta_T1 : Constant  Value=0
  CL delta_a1 : Constant  Value=0
  CL delta_e1 : Constant  Value=ae.aero.cLdelta_e
  CL delta_f1 : Constant  Value=ae.aero.cLdelta_f
  CL delta_r1 : Constant  Value=0
  CL iH1 : Constant  Value=ae.aero.cLiH
  CL1 : Constant  Value=ae.aero.cL1
  CL1_1 : Constant  Value=ae.aero.cL1
  CLa1 : Constant  Value=ae.aero.cLalpha
  CLq1 : Constant  Value=ae.aero.cLq
  CLu1 : Constant  Value=ae.aero.cLu
  CTx1 : Constant  Value=ae.aero.cTx1
  CTxu : Constant  Value=ae.aero.cTxu
  Cm alphadot : Constant  Value=ae.aero.cmalphadot
  Cm delta_T : Constant  Value=0
  Cm delta_a : Constant  Value=0
  Cm delta_e : Constant  Value=ae.aero.cmdelta_e
  Cm delta_f : Constant  Value=ae.aero.cmdelta_f
  Cm delta_r : Constant  Value=0
  Cm iH : Constant  Value=ae.aero.cMiH
  Cm1 : Constant  Value=ae.aero.cm1
  CmT alpha : Constant  Value=ae.aero.cmTalpha
  CmT1 : Constant  Value=ae.aero.cmT1
  CmTu : Constant  Value=ae.aero.cmTu
  Cma : Constant  Value=ae.aero.cmalpha
  Cmq : Constant  Value=ae.aero.cmq
  Cmu : Constant  Value=ae.aero.cmu
  DeltaAileron1 : InportShadow  Port=10
  DeltaAileron2 : InportShadow  Port=10
  DeltaElevator1 : InportShadow  Port=8
  DeltaElevator2 : InportShadow  Port=8
  DeltaFlap1 : InportShadow  Port=9
  DeltaFlap2 : InportShadow  Port=9
  DeltaRudder1 : InportShadow  Port=11
  DeltaRudder2 : InportShadow  Port=11
  Delta_Thrust1 : InportShadow  Port=12
  Delta_Thrust2 : InportShadow  Port=12
  Dynamic Pressure1 : InportShadow
  Dynamic Pressure2 : InportShadow
  Lift : Subsystem
  Linear Vel Body_1 : InportShadow  Port=3
  Linear Vel Body_2 : InportShadow  Port=3
  Pitch : Subsystem
  S_1 : InportShadow  Port=2
  S_2 : InportShadow  Port=2
  c_bar1 : InportShadow  Port=5
  c_bar2 : InportShadow  Port=5
  drag : Subsystem
  iH1 : InportShadow  Port=13
  iH2 : InportShadow  Port=13
  D : Outport  VectorParamsAs1DForOutWhenUnconnected=off
  m : Outport  Port=2  VectorParamsAs1DForOutWhenUnconnected=off
  L : Outport  Port=3  VectorParamsAs1DForOutWhenUnconnected=off
  wires:
  DeltaRudder/1 -> drag/10(Delta_r)
  DeltaAileron/1 -> drag/8(Delta_a)
  CDa/1 -> drag/17(CDa)
  Alpha/1 -> drag/5(Alpha)
  CDu/1 -> drag/14(CDu)
  Alpha_dot/1 -> drag/6(Alpha_dot)
  drag/1(Out1) -> D/1
  Lift/1(Out1) -> L/1
  S/1 -> drag/2(S)
  Dynamic Pressure/1 -> drag/1(q)
  Linear Vel Body/1 -> drag/3(Linear Vel Body)
  Delta_Thrust/1 -> drag/12(Delta_Thrust)
  iH/1 -> drag/11(iH)
  CD delta_T/1 -> drag/24(CDdelta_T)
  DeltaElevator/1 -> drag/7(Delta_e)
  DeltaFlap/1 -> drag/9(Delta_f)
  Pitch/1(Out1) -> m/1
  c_bar/1 -> drag/4(c_bar)
  CD alphadot/1 -> drag/18(CDalpha_dot)
  CDq/1 -> drag/19(CDq)
  CD delta_e/1 -> drag/20(CDdelta_e)
  CD delta_a/1 -> drag/21(CDdelta_a)
  CD delta_f/1 -> drag/22(CDdelta_f)
  CD delta_r/1 -> drag/23(CDdelta_r)
  CD iH/1 -> drag/25(CD_ih)
  CTx1/1 -> drag/15(CTx1)
  CD1/1 -> drag/13(CD1)
  CTxu/1 -> drag/16(CTxu)
  DeltaRudder1/1 -> Pitch/11(Delta_r)
  DeltaAileron1/1 -> Pitch/9(Delta_a)
  Alpha1/1 -> Pitch/6(Alpha)
  Alpha_dot1/1 -> Pitch/7(Alpha_dot)
  S_1/1 -> Pitch/2(S)
  Dynamic Pressure2/1 -> Pitch/1(q)
  Linear Vel Body_2/1 -> Pitch/3(Linear Vel Body)
  Delta_Thrust1/1 -> Pitch/13(Delta_Thrust)
  iH1/1 -> Pitch/12(iH)
  DeltaElevator1/1 -> Pitch/8(Delta_e)
  DeltaFlap1/1 -> Pitch/10(Delta_f)
  S_2/1 -> Lift/2(S)
  Dynamic Pressure1/1 -> Lift/1(q)
  Linear Vel Body_1/1 -> Lift/3(Linear Vel Body)
  Delta_Thrust2/1 -> Lift/12(Delta_Thrust)
  c_bar2/1 -> Lift/4(c_bar)
  CL1/1 -> drag/26(CL1)
  iH2/1 -> Lift/11(iH)
  DeltaRudder2/1 -> Lift/10(Delta_r)
  DeltaFlap2/1 -> Lift/9(Delta_f)
  DeltaAileron2/1 -> Lift/8(Delta_a)
  DeltaElevator2/1 -> Lift/7(Delta_e)
  Alpha_dot2/1 -> Lift/6(Alpha_dot)
  Alpha2/1 -> Lift/5(Alpha)
  Angular Vel/1 -> Pitch/4(Angular Vel)
  c_bar1/1 -> Pitch/5(c_bar)
  CD1_1/1 -> Lift/24(CD1)
  CLa1/1 -> Lift/15(CLa)
  CLq1/1 -> Lift/17(CLq)
  CL delta_a1/1 -> Lift/19(CLdelta_a)
  CL delta_r1/1 -> Lift/21(CLdelta_r)
  CL iH1/1 -> Lift/23(CL_ih)
  CL delta_T1/1 -> Lift/22(CLdelta_T)
  CLu1/1 -> Lift/14(CLu)
  CL alphadot1/1 -> Lift/16(CLalpha_dot)
  CL delta_f1/1 -> Lift/20(CLdelta_f)
  CL delta_e1/1 -> Lift/18(CLdelta_e)
  CL1_1/1 -> Lift/13(CL1)
  CmT alpha/1 -> Pitch/18(CmTa)
  Cm alphadot/1 -> Pitch/20(Cmalpha_dot)
  Cm delta_e/1 -> Pitch/22(Cmdelta_e)
  Cm delta_f/1 -> Pitch/24(Cmdelta_f)
  Cm delta_T/1 -> Pitch/26(Cmdelta_T)
  CmT1/1 -> Pitch/16(CmT1)
  Cm1/1 -> Pitch/14(Cm1)
  CmTu/1 -> Pitch/17(CmTu)
  Cmq/1 -> Pitch/21(Cmq)
  Cm delta_a/1 -> Pitch/23(Cmdelta_a)
  Cm delta_r/1 -> Pitch/25(Cmdelta_r)
  Cmu/1 -> Pitch/15(Cmu)
  Cma/1 -> Pitch/19(Cma)
  Cm iH/1 -> Pitch/27(Cm_ih)

== system NFSModelsLibrary/Forces and Moments/Gravity Calculator ==
  Position (NED) : Inport
  Flat Earth to LLA : aerolibtransform2/Flat Earth to LLA  units=Metric (MKS)  ptype=Earth (WGS84)  F=1/298.257223563  R=6378137  refPosPort=off  LL0=[nfs.Coordinate.Lat nfs.Coordinate.Long]  psi=0
  Mux1 : Mux  Inputs=2
  Ref Alt : Constant  Value=0
  Reshape : Reshape  OutputDimensionality=Customize  OutputDimensions=[1,3]
  Reshape1 : Reshape  OutputDimensionality=Customize  OutputDimensions=[3,1]
  "WGS84 Gravity Model  " : GravityWGS84
  Gravity (NED) : Outport  VectorParamsAs1DForOutWhenUnconnected=off
  Altitud : Outport  Port=2  VectorParamsAs1DForOutWhenUnconnected=off
  wires:
  Mux1/1 -> Reshape/1
  Flat Earth to LLA/2 -> Mux1/2, Altitud/1
  Reshape/1 -> "WGS84 Gravity Model  "/1
  Flat Earth to LLA/1 -> Mux1/1
  Position (NED)/1 -> Flat Earth to LLA/1
  Ref Alt/1 -> Flat Earth to LLA/2
  "WGS84 Gravity Model  "/1 -> Reshape1/1
  Reshape1/1 -> Gravity (NED)/1

== system NFSModelsLibrary/Forces and Moments/Thrust ==
  Trim Thrust : Inport
  Manual Switch : ManualSwitch  CurrentSetting=0
  Mux1 : Mux  Inputs=3
  Product : Product  RndMeth=Zero
  Product1 : Product  RndMeth=Zero
  Signal Builder : Subsystem  Tag=STV Subsys  LoadFcn=sigbuilder_block('load');  StartFcn=sigbuilder_block('start');  StopFcn=sigbuilder_block('stop');  ClipboardFcn=sigbuilder_block('clipboard');  mask(Sigbuilder block){tuvar=[0:10]}
      mask help: Simulink:masks:SigbuilderBlock_MD
      mask init:
      | if ~strcmp(get_param(bdroot(gcbh),'SimulationStatus'),'stopped') tuvar = sigbuilder_block('maskInit'); end
      settings: CopyFcn=sigbuilder_block('copy');  DeleteFcn=sigbuilder_block('delete');  ModelCloseFcn=sigbuilder_block('modelClose');  PreSaveFcn=sigbuilder_block('preSave');  PauseFcn=sigbuilder_block('pause');  ContinueFcn=sigbuilder_block('continue');  NameChangeFcn=sigbuilder_block('namechange');  OpenFcn=sigbuilder_block('open',[437.25 199.5 550.5 399.75 ]);  CloseFcn=sigbuilder_block('close');
      mask Display: plot(0, 0, 100, 100,[2, 2, 32, 32, 2], [68, 8, 8, 68, 68],[32, 2], [38, 38], [32, 19, 2],[53, 60, 44], [32, 17, 17, 2],[16, 16, 31, 31]);txt = getActiveGroup(gcbh);text(2, 100, txt,'verticalAlignment', 'top');
  Throttle : Gain
  Trim Thrust1 : Constant  Value=cos(nfs.tmisalign)
  Trim Thrust2 : Constant  Value=sin(nfs.tmisalign)
  Trim Thrust3 : Constant  Value=0
  Trim Thrust4 : Constant
  Trim Thrust5 : Constant  Value=[0;0;0]
  Thrust Force : Outport  PortDimensions=[3,1]  VectorParamsAs1DForOutWhenUnconnected=off
  Thrust Moment : Outport  Port=2  PortDimensions=[3,1]  VectorParamsAs1DForOutWhenUnconnected=off
  wires:
  Mux1/1 -> Throttle/1
  Trim Thrust3/1 -> Mux1/3
  Trim Thrust2/1 -> Mux1/2
  Trim Thrust1/1 -> Mux1/1
  Throttle/1 -> Product/1
  Product/1 -> Product1/1
  Manual Switch/1 -> Product/2
  Signal Builder/1(ThrustDeviation) -> Manual Switch/1
  Trim Thrust4/1 -> Manual Switch/2
  Trim Thrust5/1 -> Thrust Moment/1
  Trim Thrust/1 -> Product1/2
  Product1/1 -> Thrust Force/1

== system NFSModelsLibrary/Forces and Moments/Weight ==
  note: theta
  note: phi
  Attitute : Inport  PortDimensions=[3,1]
  Gravity : Inport  Port=2  PortDimensions=[3,1]
  Demux : Demux  Outputs=3
  Gain1 : Gain  Gain=-1
  Mux1 : Mux  Inputs=3
  Product{1..2,4..5} (4 alike) : Product  RndMeth=Zero
  Terminator4 : Terminator
  Trigonometric Function1 : Trigonometry  Operator=cos
  Trigonometric Function2 : Trigonometry
  Trigonometric Function3 : Trigonometry  Operator=cos
  Trigonometric Function4 : Trigonometry
  Trim Thrust5 : Constant  Value=[0;0;0]
  Vector Magnitude : Subsystem
  mass : Constant  Value=nfs.mass
  Weight Force : Outport  PortDimensions=[3,1]  VectorParamsAs1DForOutWhenUnconnected=off
  Weight Moment : Outport  Port=2  PortDimensions=[3,1]  VectorParamsAs1DForOutWhenUnconnected=off
  wires:
  Mux1/1 -> Product2/1
  Product5/1 -> Mux1/3
  Product4/1 -> Mux1/2
  Gain1/1 -> Mux1/1
  Trigonometric Function1/1 -> Product5/2
  Trigonometric Function4/1 -> Product4/1
  Trigonometric Function3/1 -> Product5/1, Product4/2
  Trigonometric Function2/1 -> Gain1/1
  mass/1 -> Product1/1
  Demux/3 -> Terminator4/1
  Attitute/1 -> Demux/1
  Demux/2 -> Trigonometric Function3/1, Trigonometric Function2/1
  Demux/1 -> Trigonometric Function1/1, Trigonometric Function4/1
  Trim Thrust5/1 -> Weight Moment/1
  Gravity/1 -> Vector Magnitude/1(Vector)
  Product1/1 -> Product2/2
  Product2/1 -> Weight Force/1
  Vector Magnitude/1(Vector Magnitude) -> Product1/2

== system NFSModelsLibrary/3-AxisAccelerometer/Accelerometer Dynamic/No Dynamics ==
  In : Inport
  Gain : Gain  Gain=0
  "Out " : Outport  VectorParamsAs1DForOutWhenUnconnected=off
  wires:
  In/1 -> Gain/1
  Gain/1 -> "Out "/1

== system NFSModelsLibrary/3-AxisAccelerometer/Accelerometer Dynamic/Second-order Dynamics ==
  In : Inport
  Demux : Demux  Outputs=3
  Mux : Mux  Inputs=3
  Transfer Fcn X : TransferFcn  Numerator=[w_a*w_a]  Denominator="[1 2*z_a*w_a  w_a*w_a]"
  Transfer Fcn Y : TransferFcn  Numerator=[w_a*w_a]  Denominator="[1 2*z_a*w_a  w_a*w_a]"
  Transfer Fcn Z : TransferFcn  Numerator=[w_a*w_a]  Denominator="[1 2*z_a*w_a  w_a*w_a]"
  "Out " : Outport  VectorParamsAs1DForOutWhenUnconnected=off
  wires:
  Transfer Fcn Y/1 -> Mux/2
  In/1 -> Demux/1
  Demux/1 -> Transfer Fcn X/1
  Transfer Fcn Z/1 -> Mux/3
  Demux/2 -> Transfer Fcn Y/1
  Demux/3 -> Transfer Fcn Z/1
  Mux/1 -> "Out "/1
  Transfer Fcn X/1 -> Mux/1

== system NFSModelsLibrary/3-AxisAccelerometer/Noise Check/No Noise ==
  In : Inport
  Gain : Gain  Gain=0
  "Out " : Outport  VectorParamsAs1DForOutWhenUnconnected=off
  wires:
  In/1 -> Gain/1
  Gain/1 -> "Out "/1

== system NFSModelsLibrary/3-AxisAccelerometer/Noise Check/Noisy Signal ==
  In : Inport
  "Out " : Outport  VectorParamsAs1DForOutWhenUnconnected=off
  wires:
  In/1 -> "Out "/1

== system NFSModelsLibrary/3-AxisRateGyro/Gyroscope Dynamic/2nd-Order Dynamics ==
  In : Inport  PortDimensions=[3,1]
  Demux : Demux  Outputs=3
  Mux : Mux  Inputs=3
  Transfer Fcn X : TransferFcn  Numerator=[w_g*w_g]  Denominator="[1 2*z_g*w_g  w_g*w_g]"
  Transfer Fcn Y : TransferFcn  Numerator=[w_g*w_g]  Denominator="[1 2*z_g*w_g  w_g*w_g]"
  Transfer Fcn Z : TransferFcn  Numerator=[w_g*w_g]  Denominator="[1 2*z_g*w_g  w_g*w_g]"
  Out : Outport  PortDimensions=[3,1]  VectorParamsAs1DForOutWhenUnconnected=off
  wires:
  In/1 -> Demux/1
  Demux/3 -> Transfer Fcn Z/1
  Demux/2 -> Transfer Fcn Y/1
  Mux/1 -> Out/1
  Transfer Fcn Y/1 -> Mux/2
  Transfer Fcn X/1 -> Mux/1
  Demux/1 -> Transfer Fcn X/1
  Transfer Fcn Z/1 -> Mux/3

== system NFSModelsLibrary/3-AxisRateGyro/Gyroscope Dynamic/No Dynamics ==
  In : Inport  PortDimensions=[3,1]
  Out : Outport  PortDimensions=[3,1]  VectorParamsAs1DForOutWhenUnconnected=off
  wires:
  In/1 -> Out/1
